simulink model "model"  (R2020b)
settings: Solver=VariableStepAuto  StartTime=0.0  StopTime=10.0  RelTol=1e-3
values from neighbouring files (symbols this model uses):
  be = 2.0    [clutch_lockup_data.sldd]
  bv = 1.0    [clutch_lockup_data.sldd]
  Ie = 1.0    [clutch_lockup_data.sldd]
  Iv = 5.0    [clutch_lockup_data.sldd]
  muk = 1.0    [clutch_lockup_data.sldd]
  mus = 1.5    [clutch_lockup_data.sldd]
  R = 1.0    [clutch_lockup_data.sldd]
settings Model: Creator=Pavan  LastModifiedBy=Pavan

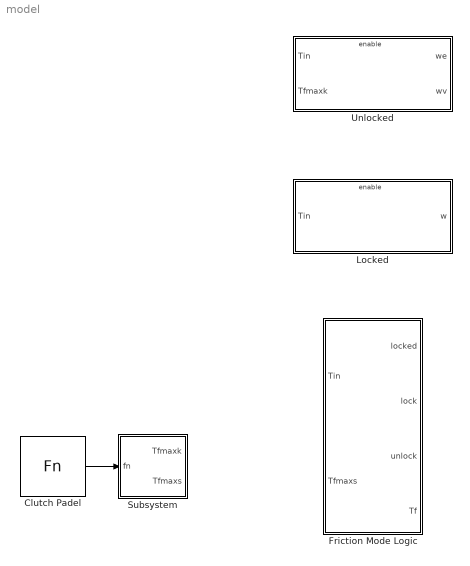
== system model ==
  Clutch Padel : FromWorkspace  VariableName=Fn
  Friction Mode Logic : Subsystem
  Locked : Subsystem
  Subsystem : Subsystem
  Unlocked : Subsystem
  wires:
  Clutch Padel/1 -> Subsystem/1(fn)

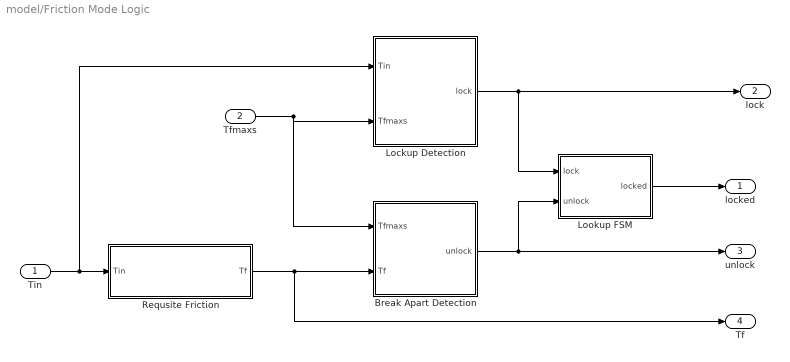
== system model/Friction Mode Logic ==
  Tin : Inport
  Tfmaxs : Inport  Port=2
  Break Apart Detection : Subsystem
  Lockup Detection : Subsystem
  Lookup FSM : Subsystem
  Requsite Friction : Subsystem
  locked : Outport
  lock : Outport  Port=2
  unlock : Outport  Port=3
  Tf : Outport  Port=4
  wires:
  Requsite Friction/1(Tf) -> Tf/1, Break Apart Detection/2(Tf)
  Lookup FSM/1(locked) -> locked/1
  Tfmaxs/1 -> Break Apart Detection/1(Tfmaxs), Lockup Detection/2(Tfmaxs)
  Break Apart Detection/1(unlock) -> unlock/1, Lookup FSM/2(unlock)
  Tin/1 -> Lockup Detection/1(Tin), Requsite Friction/1(Tin)
  Lockup Detection/1(lock) -> lock/1, Lookup FSM/1(lock)

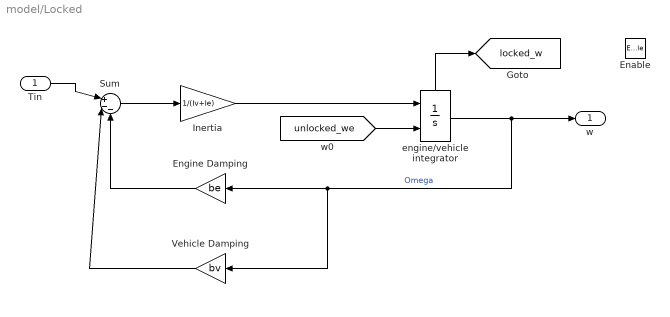
== system model/Locked ==
  Tin : Inport
  Enable : EnablePort
  Engine Damping : Gain  Gain=be
  Inertia : Gain  Gain=1/(Iv+Ie)
  Sum : Sum  Inputs=|+--
  Vehicle Damping : Gain  Gain=bv
  engine/vehicle integrator : Integrator  InitialConditionSource=external  ShowStatePort=on
  w : Outport
  tag scope: locked_w=global
  wires:
  Engine Damping/1 -> Sum/3
  Sum/1 -> Inertia/1
  engine/vehicle integrator/1 -> w/1, Vehicle Damping/1, Engine Damping/1  "Omega"
  [unlocked_we] -> engine/vehicle integrator/2
  Inertia/1 -> engine/vehicle integrator/1
  Vehicle Damping/1 -> Sum/2
  engine/vehicle integrator/State -> [locked_w]
  Tin/1 -> Sum/1

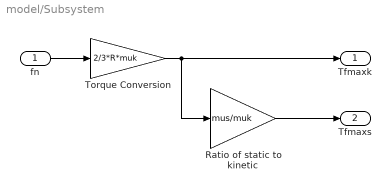
== system model/Subsystem ==
  fn : Inport
  Ratio of static to kinetic : Gain  Gain=mus/muk
  Torque Conversion : Gain  Gain=2/3*R*muk
  Tfmaxk : Outport
  Tfmaxs : Outport  Port=2
  wires:
  Torque Conversion/1 -> Tfmaxk/1, Ratio of static to kinetic/1
  fn/1 -> Torque Conversion/1
  Ratio of static to kinetic/1 -> Tfmaxs/1

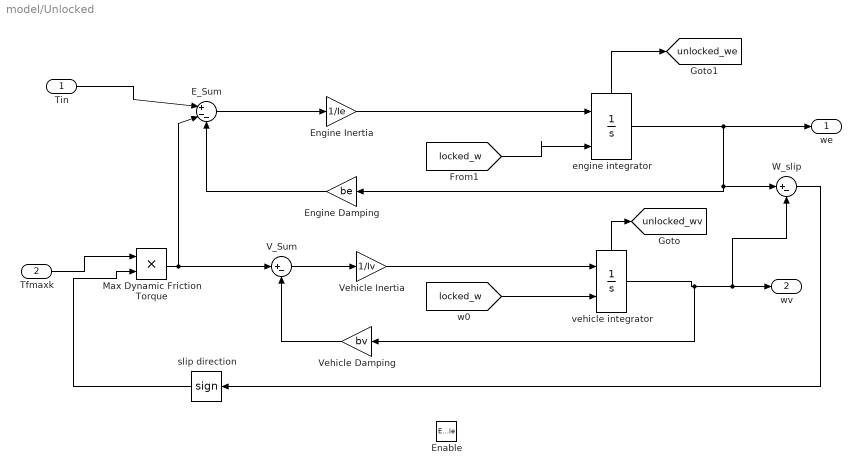
== system model/Unlocked ==
  Tin : Inport
  Tfmaxk : Inport  Port=2
  Enable : EnablePort
  E_Sum : Sum  Inputs=|+--
  Engine Damping : Gain  Gain=be
  Engine Inertia : Gain  Gain=1/Ie
  Max Dynamic Friction Torque : Product
  V_Sum : Sum  Inputs=|+-
  Vehicle Damping : Gain  Gain=bv
  Vehicle Inertia : Gain  Gain=1/Iv
  W_slip : Sum  Inputs=|+-
  engine integrator : Integrator  InitialConditionSource=external  ShowStatePort=on
  slip direction : Signum
  vehicle integrator : Integrator  InitialConditionSource=external  ShowStatePort=on
  we : Outport
  wv : Outport  Port=2
  tag scope: unlocked_we=global, unlocked_wv=global
  wires:
  Engine Inertia/1 -> engine integrator/1
  V_Sum/1 -> Vehicle Inertia/1
  vehicle integrator/1 -> wv/1, W_slip/2, Vehicle Damping/1
  [locked_w] -> vehicle integrator/2
  engine integrator/1 -> we/1, W_slip/1, Engine Damping/1
  [locked_w] -> engine integrator/2
  vehicle integrator/State -> [unlocked_wv]
  engine integrator/State -> [unlocked_we]
  Max Dynamic Friction Torque/1 -> V_Sum/1, E_Sum/2
  Tfmaxk/1 -> Max Dynamic Friction Torque/1
  Engine Damping/1 -> E_Sum/3
  Tin/1 -> E_Sum/1
  E_Sum/1 -> Engine Inertia/1
  Vehicle Inertia/1 -> vehicle integrator/1
  slip direction/1 -> Max Dynamic Friction Torque/2
  Vehicle Damping/1 -> V_Sum/2
  W_slip/1 -> slip direction/1

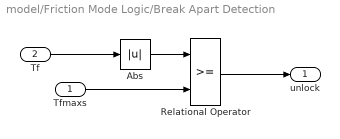
== system model/Friction Mode Logic/Break Apart Detection ==
  Tfmaxs : Inport
  Tf : Inport  Port=2
  Abs : Abs
  Relational Operator : RelationalOperator  OutDataTypeStr=boolean  RndMeth=Simplest
  unlock : Outport
  wires:
  Relational Operator/1 -> unlock/1
  Tf/1 -> Abs/1
  Abs/1 -> Relational Operator/1
  Tfmaxs/1 -> Relational Operator/2

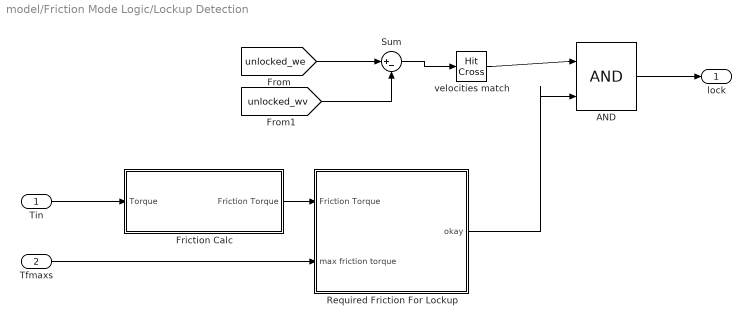
== system model/Friction Mode Logic/Lockup Detection ==
  Tin : Inport
  Tfmaxs : Inport  Port=2
  AND : Logic  IconShape=distinctive  AllPortsSameDT=off  OutDataTypeStr=boolean
  Friction Calc : Subsystem
  Required Friction For Lockup : Subsystem
  Sum : Sum  Inputs=|+-
  velocities match : HitCross
  lock : Outport
  wires:
  Tfmaxs/1 -> Required Friction For Lockup/2(max friction torque)
  Friction Calc/1(Friction Torque) -> Required Friction For Lockup/1(Friction Torque)
  velocities match/1 -> AND/1
  Sum/1 -> velocities match/1
  AND/1 -> lock/1
  Required Friction For Lockup/1(okay) -> AND/2
  Tin/1 -> Friction Calc/1(Torque)
  [unlocked_wv] -> Sum/2
  [unlocked_we] -> Sum/1

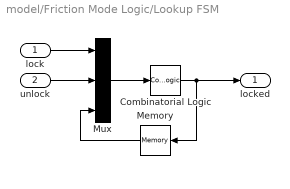
== system model/Friction Mode Logic/Lookup FSM ==
  lock : Inport
  unlock : Inport  Port=2
  Combinatorial Logic : CombinatorialLogic  TruthTable=[0;1;0;0;1;1;1;0]
  Memory : Memory
  Mux : Mux  Inputs=3
  locked : Outport
  wires:
  unlock/1 -> Mux/2
  Mux/1 -> Combinatorial Logic/1
  Combinatorial Logic/1 -> locked/1, Memory/1
  Memory/1 -> Mux/3
  lock/1 -> Mux/1

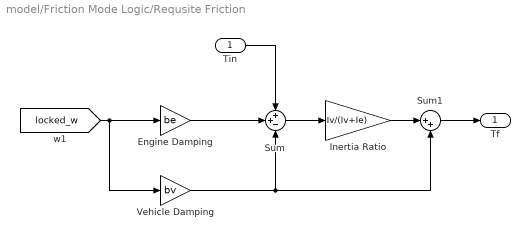
== system model/Friction Mode Logic/Requsite Friction ==
  Tin : Inport
  Engine Damping : Gain  Gain=be
  Inertia Ratio : Gain  Gain=Iv/(Iv+Ie)
  Sum : Sum  Inputs=++-
  Sum1 : Sum  Inputs=|++
  Vehicle Damping : Gain  Gain=bv
  Tf : Outport
  wires:
  Inertia Ratio/1 -> Sum1/1
  [locked_w] -> Vehicle Damping/1, Engine Damping/1
  Sum/1 -> Inertia Ratio/1
  Engine Damping/1 -> Sum/2
  Vehicle Damping/1 -> Sum1/2, Sum/3
  Tin/1 -> Sum/1
  Sum1/1 -> Tf/1

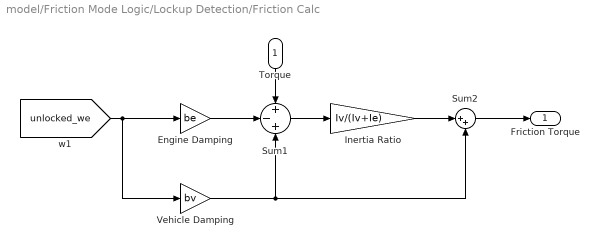
== system model/Friction Mode Logic/Lockup Detection/Friction Calc ==
  Torque : Inport
  Engine Damping : Gain  Gain=be
  Inertia Ratio : Gain  Gain=Iv/(Iv+Ie)
  Sum1 : Sum  Inputs=+-+
  Sum2 : Sum  Inputs=|++
  Vehicle Damping : Gain  Gain=bv
  Friction Torque : Outport
  wires:
  Sum1/1 -> Inertia Ratio/1
  Sum2/1 -> Friction Torque/1
  Vehicle Damping/1 -> Sum2/2, Sum1/3
  [unlocked_we] -> Vehicle Damping/1, Engine Damping/1
  Engine Damping/1 -> Sum1/2
  Torque/1 -> Sum1/1
  Inertia Ratio/1 -> Sum2/1

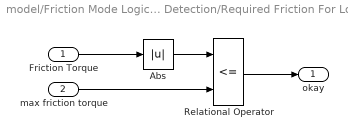
== system model/Friction Mode Logic/Lockup Detection/Required Friction For Lockup ==
  Friction Torque : Inport
  max friction torque : Inport  Port=2
  Abs : Abs
  Relational Operator : RelationalOperator  Operator=<=  OutDataTypeStr=boolean  RndMeth=Simplest
  okay : Outport
  wires:
  Relational Operator/1 -> okay/1
  Friction Torque/1 -> Abs/1
  max friction torque/1 -> Relational Operator/2
  Abs/1 -> Relational Operator/1
